simulink model "simulacionPIDv2"  (R2020a)
settings: Solver=FixedStepAuto  StartTime=0.0  StopTime=15.0  FixedStep=0.01  RelTol=1e-3
undefined symbols (not defined in the file): Fden2, Fnum2, PIDden, PIDnum, tf_6polos_num, tf_polos_den
settings Model: Creator=nacho  LastModifiedBy=nacho

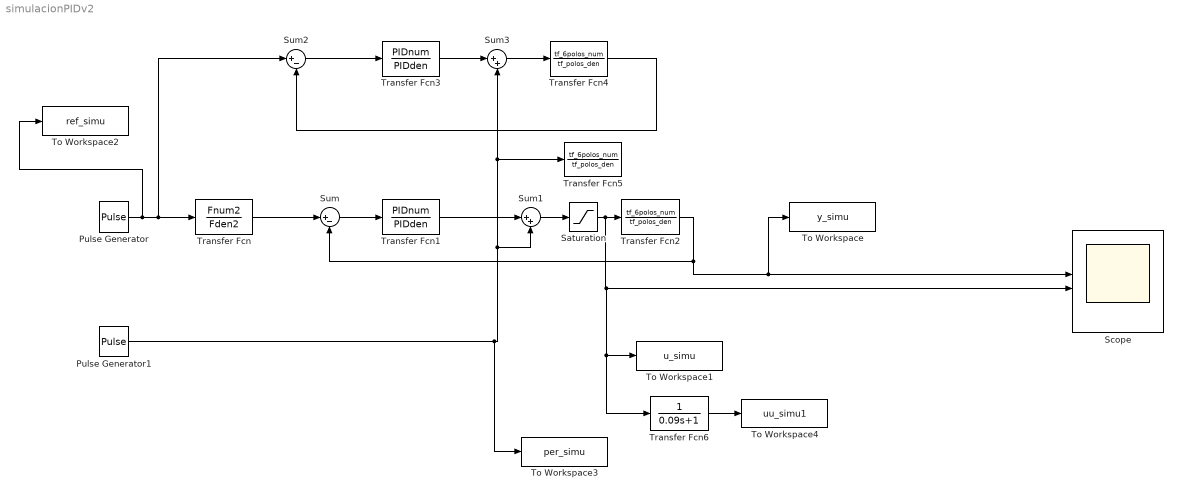
== system simulacionPIDv2 ==
  Pulse Generator : DiscretePulseGenerator  PulseType=Time based  Amplitude=3  Period=20  PulseWidth=50  PhaseDelay=1
  Pulse Generator1 : DiscretePulseGenerator  PulseType=Time based  Amplitude=-1  Period=100  PulseWidth=50  PhaseDelay=6
  Saturation : Saturate  UpperLimit=4  LowerLimit=-1
  Scope : Scope  NumInputPorts=6
  Sum : Sum  Inputs=|+-
  Sum1 : Sum  Inputs=|++
  Sum2 : Sum  Inputs=|+-
  Sum3 : Sum  Inputs=|++
  To Workspace : ToWorkspace  VariableName=y_simu  SaveFormat=Timeseries  SampleTime=-1
  To Workspace1 : ToWorkspace  VariableName=u_simu  SaveFormat=Timeseries  SampleTime=-1
  To Workspace2 : ToWorkspace  VariableName=ref_simu  SaveFormat=Timeseries  SampleTime=-1
  To Workspace3 : ToWorkspace  VariableName=per_simu  SaveFormat=Timeseries  SampleTime=-1
  To Workspace4 : ToWorkspace  VariableName=uu_simu1  SaveFormat=Timeseries  SampleTime=-1
  Transfer Fcn : TransferFcn  Numerator=Fnum2  Denominator=Fden2
  Transfer Fcn1 : TransferFcn  Numerator=PIDnum  Denominator=PIDden
  Transfer Fcn2 : TransferFcn  Numerator=tf_6polos_num  Denominator=tf_polos_den
  Transfer Fcn3 : TransferFcn  Numerator=PIDnum  Denominator=PIDden
  Transfer Fcn4 : TransferFcn  Numerator=tf_6polos_num  Denominator=tf_polos_den
  Transfer Fcn5 : TransferFcn  Numerator=tf_6polos_num  Denominator=tf_polos_den
  Transfer Fcn6 : TransferFcn  Denominator=[0.09 1]
  wires:
  Sum/1 -> Transfer Fcn1/1
  Transfer Fcn/1 -> Sum/1
  Transfer Fcn2/1 -> Sum/2, To Workspace/1, Scope/3
  Pulse Generator/1 -> To Workspace2/1, Sum2/1, Transfer Fcn/1
  Pulse Generator1/1 -> To Workspace3/1, Sum1/2, Transfer Fcn5/1, Sum3/2
  Transfer Fcn3/1 -> Sum3/1
  Transfer Fcn4/1 -> Sum2/2
  Sum2/1 -> Transfer Fcn3/1
  Sum3/1 -> Transfer Fcn4/1
  Transfer Fcn1/1 -> Sum1/1
  Sum1/1 -> Saturation/1
  Saturation/1 -> Transfer Fcn6/1, To Workspace1/1, Scope/4, Transfer Fcn2/1
  Transfer Fcn6/1 -> To Workspace4/1
